simulink model "simulink_group17f"  (R2024a)
settings: Solver=FixedStepDiscrete  StartTime=0.0  StopTime=10.0  FixedStep=1e-3  RelTol=1e-3  EnableMultiTasking=on
undefined symbols (not defined in the file): A0, A1, D0, D1, D10, D11, D12, D13, D2, D3, D4, D5, D6, D7, D8, D9, PTA0, PTA1, PTA2, PTB2, PTB23, PTB3, PTB9, PTC16, PTC17, PTC2, PTC3, PTC4, PTD0, PTD1, PTD2, PTD3
libraries: frdmk64flib x20, dspstat3 x1, simulink x1
settings Model: ExtModeTrigDuration=5  Creator=ow  LastModifiedBy=furqa
settings SolverCC: AlgebraicLoopSolver=TrustRegion
settings OptimizationCC: EnhancedBackFolding=on  PassReuseOutputArgsAs=Individual arguments  ZeroExternalMemoryAtStartup=off  ZeroInternalMemoryAtStartup=off  MaxStackSize=64  OptimizeBlockOrder=speed  DifferentSizesBufferReuse=on  OptimizationCustomize=off  EfficientTunableParamExpr=on
settings DebuggingCC: ParameterTunabilityLossMsg=error  UnconnectedInputMsg=warning  UnconnectedOutputMsg=warning  UnconnectedLineMsg=warning
settings HardwareCC: ProdBitPerPointer=32  ProdBitPerSizeT=32  ProdBitPerPtrDiffT=32  ProdLargestAtomicInteger=Long  ProdLargestAtomicFloat=Double  ProdWordSize=32  ProdHWDeviceType=ARM Compatible->ARM Cortex
settings ModelReferenceCC: EnableRefExpFcnMdlSchedulingChecks=on
settings SFSimCC: MATLABDynamicMemAlloc=off
settings RTWCC: Description=Embedded Coder  SystemTargetFile=ert.tlc  HardwareBoard=NXP FRDM-K64F  TLCOptions="-aInlineSetEventsForThisBaseRateFcn=TLC_FALSE -aSuppressMultiTaskScheduler=TLC_FALSE  -aRateBasedStepFcn=0"  TemplateMakefile=ert_default_tmf  Toolchain=GNU Tools for ARM Embedded Processors  GPUComputeCapability=3.5
settings CodeAppCC: ForceParamTrailComments=on  IgnoreCustomStorageClasses=off  OperatorAnnotations=on  SimulinkDataObjDesc=on  SFDataObjDesc=on  InsertBlockDesc=on

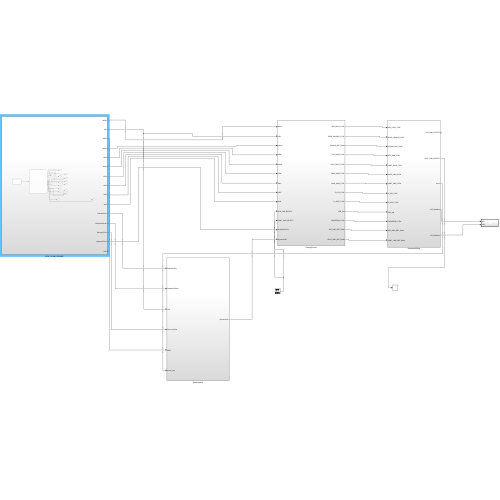
[thumbnail: Simulink's stored preview of the top-level diagram]
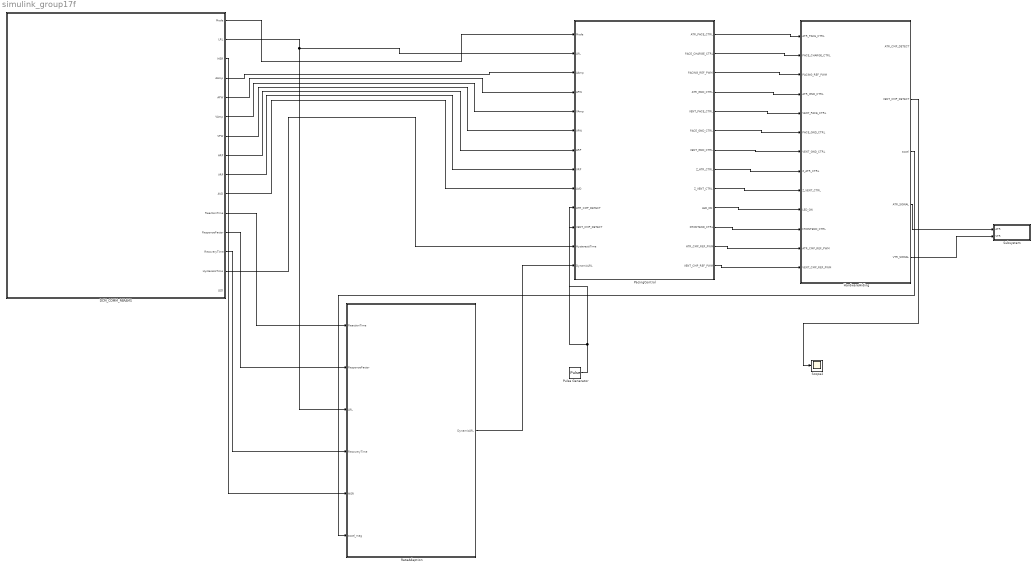
== system simulink_group17f ==
  DCM_COMM_PARAMS : Subsystem
  HardwareHiding : Subsystem
  PacingControl : Subsystem
  Pulse Generator : DiscretePulseGenerator  Period=600  PulseWidth=5  SampleTime=0.001
  RateAdaption : Subsystem
  Scope2 : Scope
  Subsystem : Subsystem  TreatAsAtomicUnit=on  SystemSampleTime=0.01
  wires:
  HardwareHiding/3(accel) -> RateAdaption/6(accel_mag)
  PacingControl/1(ATR_PACE_CTRL) -> HardwareHiding/1(ATR_PACE_CTRL)
  PacingControl/2(PACE_CHARGE_CTRL) -> HardwareHiding/2(PACE_CHARGE_CTRL)
  PacingControl/3(PACING_REF_PWM) -> HardwareHiding/3(PACING_REF_PWM)
  PacingControl/4(ATR_GND_CTRL) -> HardwareHiding/4(ATR_GND_CTRL)
  PacingControl/5(VENT_PACE_CTRL) -> HardwareHiding/5(VENT_PACE_CTRL)
  PacingControl/6(PACE_GND_CTRL) -> HardwareHiding/6(PACE_GND_CTRL)
  PacingControl/7(VENT_GND_CTRL) -> HardwareHiding/7(VENT_GND_CTRL)
  PacingControl/8(Z_ATR_CTRL) -> HardwareHiding/8(Z_ATR_CTRL)
  PacingControl/9(Z_VENT_CTRL) -> HardwareHiding/9(Z_VENT_CTRL)
  PacingControl/10(LED_ON) -> HardwareHiding/10(LED_ON)
  PacingControl/11(FRONTEND_CTRL) -> HardwareHiding/11(FRONTEND_CTRL)
  PacingControl/12(ATR_CMP_REF_PWM) -> HardwareHiding/12(ATR_CMP_REF_PWM)
  PacingControl/13(VENT_CMP_REF_PWM) -> HardwareHiding/13(VENT_CMP_REF_PWM)
  RateAdaption/1(DynamicLRL) -> PacingControl/13(DynamicLRL)
  HardwareHiding/2(VENT_CMP_DETECT) -> Scope2/1
  Pulse Generator/1 -> PacingControl/10(ATR_CMP_DETECT), PacingControl/11(VENT_CMP_DETECT)
  DCM_COMM_PARAMS/1(Mode) -> PacingControl/1(Mode)
  DCM_COMM_PARAMS/2(LRL) -> RateAdaption/3(LRL), PacingControl/2(LRL)
  DCM_COMM_PARAMS/3(MSR) -> RateAdaption/5(MSR)
  DCM_COMM_PARAMS/4(AAmp) -> PacingControl/3(AAmp)
  DCM_COMM_PARAMS/5(APW) -> PacingControl/4(APW)
  DCM_COMM_PARAMS/6(VAmp) -> PacingControl/5(VAmp)
  DCM_COMM_PARAMS/7(VPW) -> PacingControl/6(VPW)
  DCM_COMM_PARAMS/8(ARP) -> PacingControl/7(ARP)
  DCM_COMM_PARAMS/9(VRP) -> PacingControl/8(VRP)
  DCM_COMM_PARAMS/10(AVD) -> PacingControl/9(AVD)
  DCM_COMM_PARAMS/14(HysteresisTime) -> PacingControl/12(HysteresisTime)
  DCM_COMM_PARAMS/11(ReactionTime) -> RateAdaption/1(ReactionTime)
  DCM_COMM_PARAMS/12(ResponseFactor) -> RateAdaption/2(ResponseFactor)
  DCM_COMM_PARAMS/13(RecoveryTime) -> RateAdaption/4(RecoveryTime)
  HardwareHiding/4(ATR_SIGNAL) -> Subsystem/1(ATR)
  HardwareHiding/5(VTR_SIGNAL) -> Subsystem/2(VTR)

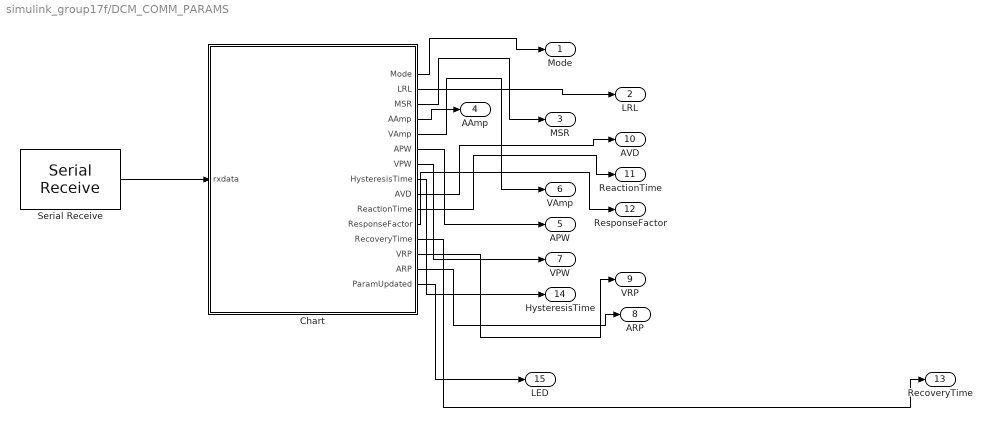
== system simulink_group17f/DCM_COMM_PARAMS ==
  Chart : Stateflow chart  TreatAsAtomicUnit=on
  Serial Receive : frdmk64flib/Serial Receive  SCIModule=0  Baudrate=uint32(9600)  Parity=None  StopBits=1  HardwareFlowControl=None  ByteOrder=LittleEndian  DataType=uint8  DataLength=31  BlockingMode=off  OutputStatus=off  SampleTime=0.001
  Mode : Outport
  LRL : Outport  Port=2
  MSR : Outport  Port=3
  AAmp : Outport  Port=4
  APW : Outport  Port=5
  VAmp : Outport  Port=6
  VPW : Outport  Port=7
  ARP : Outport  Port=8
  VRP : Outport  Port=9
  AVD : Outport  Port=10
  ReactionTime : Outport  Port=11
  ResponseFactor : Outport  Port=12
  RecoveryTime : Outport  Port=13
  HysteresisTime : Outport  Port=14
  LED : Outport  Port=15
  wires:
  Chart/1(Mode) -> Mode/1
  Chart/3(MSR) -> MSR/1
  Chart/4(AAmp) -> AAmp/1
  Chart/5(VAmp) -> VAmp/1
  Chart/6(APW) -> APW/1
  Chart/7(VPW) -> VPW/1
  Chart/8(HysteresisTime) -> HysteresisTime/1
  Chart/9(AVD) -> AVD/1
  Chart/10(ReactionTime) -> ReactionTime/1
  Chart/11(ResponseFactor) -> ResponseFactor/1
  Chart/13(VRP) -> VRP/1
  Chart/14(ARP) -> ARP/1
  Chart/2(LRL) -> LRL/1
  Chart/12(RecoveryTime) -> RecoveryTime/1
  Serial Receive/1 -> Chart/1(rxdata)
  Chart/15(ParamUpdated) -> LED/1

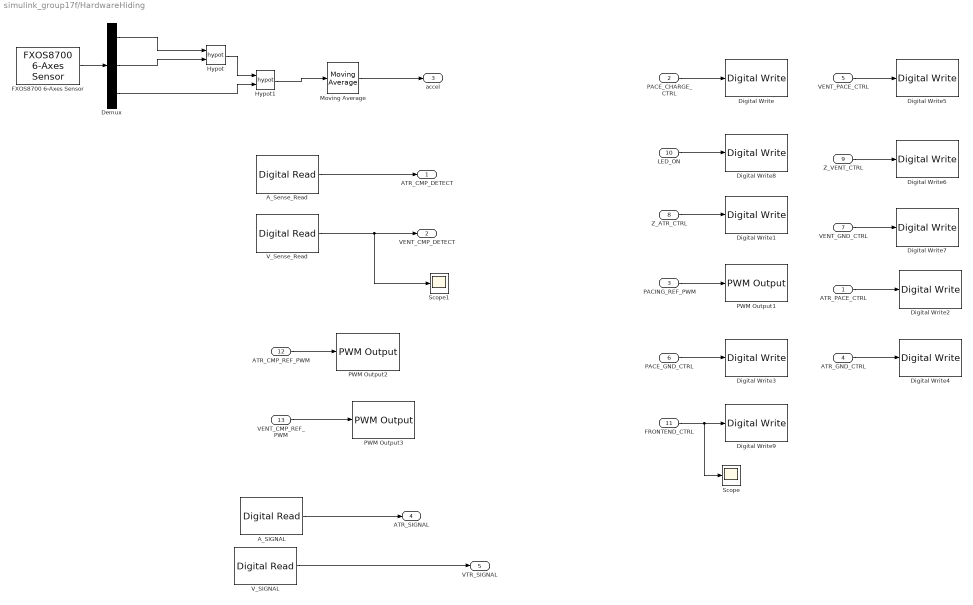
== system simulink_group17f/HardwareHiding ==
  ATR_PACE_CTRL : Inport
  PACE_CHARGE_CTRL : Inport  Port=2
  PACING_REF_PWM : Inport  Port=3
  ATR_GND_CTRL : Inport  Port=4
  VENT_PACE_CTRL : Inport  Port=5
  PACE_GND_CTRL : Inport  Port=6
  VENT_GND_CTRL : Inport  Port=7
  Z_ATR_CTRL : Inport  Port=8
  Z_VENT_CTRL : Inport  Port=9
  LED_ON : Inport  Port=10
  FRONTEND_CTRL : Inport  Port=11
  ATR_CMP_REF_PWM : Inport  Port=12
  VENT_CMP_REF_PWM : Inport  Port=13
  A_SIGNAL : frdmk64flib/Digital Read  Whichpin=PTB2 (A0)  SampleTime=0.01
  A_Sense_Read : frdmk64flib/Digital Read  Whichpin=PTC16 (D0)  SampleTime=-1
  Demux : Demux  Outputs=3
  Digital Write : frdmk64flib/Digital Write  Whichpin=PTB9 (D2)
  Digital Write1 : frdmk64flib/Digital Write  Whichpin=PTB23 (D4)
  Digital Write2 : frdmk64flib/Digital Write  Whichpin=PTA0 (D8)
  Digital Write3 : frdmk64flib/Digital Write  Whichpin=PTD0 (D10)
  Digital Write4 : frdmk64flib/Digital Write  Whichpin=PTD2 (D11)
  Digital Write5 : frdmk64flib/Digital Write  Whichpin=PTC4 (D9)
  Digital Write6 : frdmk64flib/Digital Write  Whichpin=PTC3 (D7)
  Digital Write7 : frdmk64flib/Digital Write  Whichpin=PTD3 (D12)
  Digital Write8 : frdmk64flib/Digital Write  Whichpin=RED_LED
  Digital Write9 : frdmk64flib/Digital Write  Whichpin=PTD1 (D13)
  FXOS8700 6-Axes Sensor : frdmk64flib/FXOS8700 6-Axes Sensor  Activesensor=Accelerometer only  ODR=800Hz  HybridODR=400Hz  Accelfullrange=-4g to +4g  SampleTime=-1
  Hypot : Math  Operator=hypot
  Hypot1 : Math  Operator=hypot
  Moving Average : dspstat3/Moving Average  Method=Sliding window  ForgettingFactorPort=off  SpecifyWindowLength=on  WindowLength=4  OverlapLength=3  AllowArbitraryInputLength=off  ForgettingFactor=0.9  SimulateUsing=Interpreted execution
  PWM Output1 : frdmk64flib/PWM Output  Whichpin=PTA2 (D5)  InitialFrequency=2000  InitialDutyCycle=50
  PWM Output2 : frdmk64flib/PWM Output  Whichpin=PTC2 (D6)  InitialFrequency=2000  InitialDutyCycle=100
  PWM Output3 : frdmk64flib/PWM Output  Whichpin=PTA1 (D3)  InitialFrequency=2000  InitialDutyCycle=100
  Scope : Scope
  Scope1 : Scope
  V_SIGNAL : frdmk64flib/Digital Read  Whichpin=PTB3 (A1)  SampleTime=0.01
  V_Sense_Read : frdmk64flib/Digital Read  Whichpin=PTC17 (D1)  SampleTime=-1
  ATR_CMP_DETECT : Outport
  VENT_CMP_DETECT : Outport  Port=2
  accel : Outport  Port=3
  ATR_SIGNAL : Outport  Port=4
  VTR_SIGNAL : Outport  Port=5
  wires:
  V_Sense_Read/1 -> Scope1/1, VENT_CMP_DETECT/1
  Z_VENT_CTRL/1 -> Digital Write6/1
  LED_ON/1 -> Digital Write8/1
  ATR_PACE_CTRL/1 -> Digital Write2/1
  Z_ATR_CTRL/1 -> Digital Write1/1
  VENT_GND_CTRL/1 -> Digital Write7/1
  PACE_CHARGE_CTRL/1 -> Digital Write/1
  PACE_GND_CTRL/1 -> Digital Write3/1
  PACING_REF_PWM/1 -> PWM Output1/1
  VENT_PACE_CTRL/1 -> Digital Write5/1
  ATR_GND_CTRL/1 -> Digital Write4/1
  FRONTEND_CTRL/1 -> Scope/1, Digital Write9/1
  ATR_CMP_REF_PWM/1 -> PWM Output2/1
  VENT_CMP_REF_PWM/1 -> PWM Output3/1
  Demux/1 -> Hypot/1
  Demux/2 -> Hypot/2
  Hypot/1 -> Hypot1/1
  Demux/3 -> Hypot1/2
  Hypot1/1 -> Moving Average/1
  Moving Average/1 -> accel/1
  A_Sense_Read/1 -> ATR_CMP_DETECT/1
  FXOS8700 6-Axes Sensor/1 -> Demux/1
  A_SIGNAL/1 -> ATR_SIGNAL/1
  V_SIGNAL/1 -> VTR_SIGNAL/1

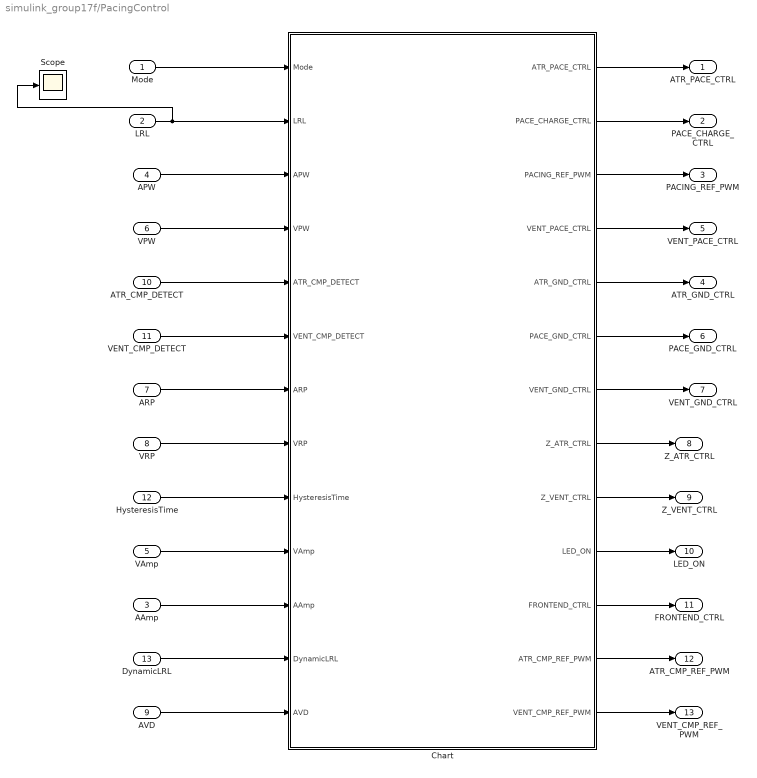
== system simulink_group17f/PacingControl ==
  Mode : Inport
  LRL : Inport  Port=2
  AAmp : Inport  Port=3
  APW : Inport  Port=4
  VAmp : Inport  Port=5
  VPW : Inport  Port=6
  ARP : Inport  Port=7
  VRP : Inport  Port=8
  AVD : Inport  Port=9
  ATR_CMP_DETECT : Inport  Port=10
  VENT_CMP_DETECT : Inport  Port=11
  HysteresisTime : Inport  Port=12
  DynamicLRL : Inport  Port=13
  Chart : Stateflow chart  TreatAsAtomicUnit=on
      settings: PortSchema="{\"entries\":[{\"content\":{\"sides\":[{\"content\":{\"connectorIds\":[\"In1\",\"In2\",\"In5\",\"In3\",\"In4\",\"In6\",\"In7\",\"In10\",\"In11\",\"In8\",\"In9\",\"In12\",\"In13\"]},\"type\":\"ConnectorPlacement.EquallySpacedRectSide\",\"uuid\":\"2cabd690-10ca-439e-b217-62815d125176\"},{\"content\":{\"connectorIds\":[\"Out1\",\"Out2\",\"Out3\",\"Out4\",\"Out5\",\"Out6\",\"Out7\",\"Out8\",\"Out9\",\"Out10\",\"Out11\",\"Out12\",\"Out13\"],\"side\":\"RIGHT\"},\"type\":\"ConnectorPlacement.EquallySpacedRectSide\",\"uuid\":\"e8964e9d-7b02-47f5-a48a-30c87640778e\"},{\"content\":{\"side\":\"TOP\"},\"type\":\"ConnectorPlacement.EquallySpacedRectSide\",\"uuid\":\"37da63f5-52a1-4b9c-b728-2e179414b5fa\"}]},\"type\":\"ConnectorPlacement.EquallySpacedConnector\",\"uuid\":\"fe4480b5-e88f-4b9f-8d05-cd2d47a8a31d\"}],\"packageUris\":[\"http://schema.mathworks.com/mf0/Connector/R2020b\"],\"version\":\"1.0\"}"
  Scope : Scope
  ATR_PACE_CTRL : Outport
  PACE_CHARGE_CTRL : Outport  Port=2
  PACING_REF_PWM : Outport  Port=3
  ATR_GND_CTRL : Outport  Port=4
  VENT_PACE_CTRL : Outport  Port=5
  PACE_GND_CTRL : Outport  Port=6
  VENT_GND_CTRL : Outport  Port=7
  Z_ATR_CTRL : Outport  Port=8
  Z_VENT_CTRL : Outport  Port=9
  LED_ON : Outport  Port=10
  FRONTEND_CTRL : Outport  Port=11
  ATR_CMP_REF_PWM : Outport  Port=12
  VENT_CMP_REF_PWM : Outport  Port=13
  wires:
  Mode/1 -> Chart/1(Mode)
  VPW/1 -> Chart/3(VPW)
  ATR_CMP_DETECT/1 -> Chart/4(ATR_CMP_DETECT)
  APW/1 -> Chart/5(APW)
  ARP/1 -> Chart/7(ARP)
  VRP/1 -> Chart/10(VRP)
  AAmp/1 -> Chart/9(AAmp)
  VAmp/1 -> Chart/8(VAmp)
  Chart/1(ATR_PACE_CTRL) -> ATR_PACE_CTRL/1
  Chart/2(PACE_CHARGE_CTRL) -> PACE_CHARGE_CTRL/1
  Chart/3(PACING_REF_PWM) -> PACING_REF_PWM/1
  Chart/5(ATR_GND_CTRL) -> ATR_GND_CTRL/1
  Chart/6(PACE_GND_CTRL) -> PACE_GND_CTRL/1
  Chart/7(VENT_GND_CTRL) -> VENT_GND_CTRL/1
  Chart/8(Z_ATR_CTRL) -> Z_ATR_CTRL/1
  Chart/9(Z_VENT_CTRL) -> Z_VENT_CTRL/1
  Chart/11(FRONTEND_CTRL) -> FRONTEND_CTRL/1
  HysteresisTime/1 -> Chart/11(HysteresisTime)
  Chart/4(VENT_PACE_CTRL) -> VENT_PACE_CTRL/1
  Chart/10(LED_ON) -> LED_ON/1
  VENT_CMP_DETECT/1 -> Chart/6(VENT_CMP_DETECT)
  Chart/12(ATR_CMP_REF_PWM) -> ATR_CMP_REF_PWM/1
  Chart/13(VENT_CMP_REF_PWM) -> VENT_CMP_REF_PWM/1
  AVD/1 -> Chart/13(AVD)
  LRL/1 -> Scope/1, Chart/2(LRL)
  DynamicLRL/1 -> Chart/12(DynamicLRL)

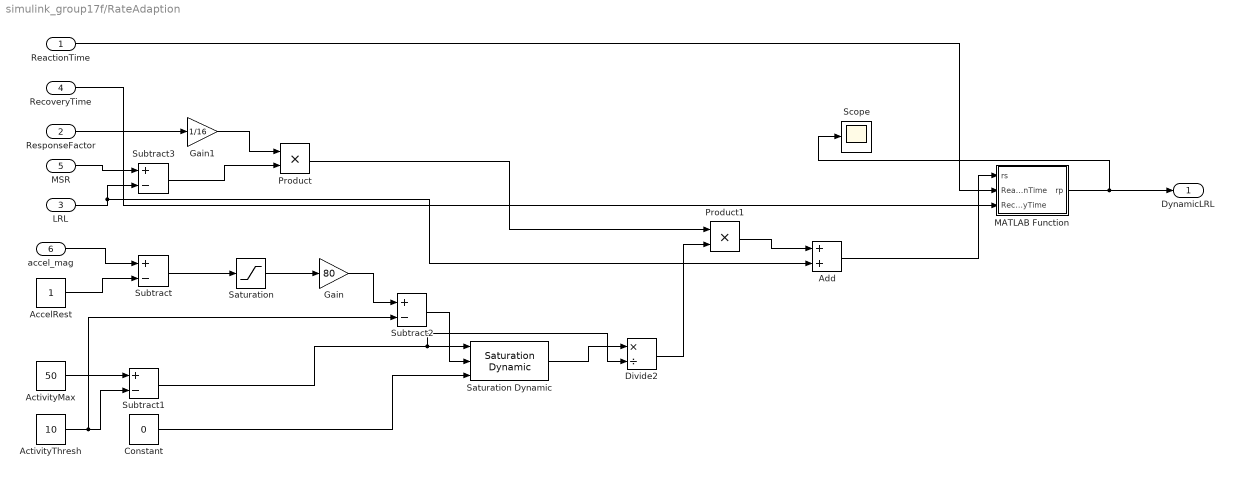
== system simulink_group17f/RateAdaption ==
  ReactionTime : Inport
  ResponseFactor : Inport  Port=2
  LRL : Inport  Port=3
  RecoveryTime : Inport  Port=4
  MSR : Inport  Port=5
  accel_mag : Inport  Port=6
  AccelRest : Constant
  ActivityMax : Constant  Value=50
  ActivityThresh : Constant  Value=10
  Add : Sum
  Constant : Constant  Value=0
  Divide2 : Product  Inputs=*/
  Gain : Gain  Gain=80
  Gain1 : Gain  Gain=1/16
  MATLAB Function : MATLAB Function  TreatAsAtomicUnit=on
  Product : Product
  Product1 : Product
  Saturation : Saturate  UpperLimit=1  LowerLimit=0
  Saturation Dynamic : simulink/Discontinuities/Saturation Dynamic  OutMin=[]  OutMax=[]  OutDataTypeStr=Inherit: Same as second input  OutDataType=fixdt(1, 16)  OutScaling=2^-10  DoSatur=off
  Scope : Scope
  Subtract{,1..3} (4 alike) : Sum  Inputs=+-
  DynamicLRL : Outport
  wires:
  accel_mag/1 -> Subtract/1
  AccelRest/1 -> Subtract/2
  Subtract/1 -> Saturation/1
  Saturation/1 -> Gain/1
  ActivityMax/1 -> Subtract1/1
  Subtract1/1 -> Divide2/2, Saturation Dynamic/1
  Gain/1 -> Subtract2/1
  Subtract2/1 -> Saturation Dynamic/2
  Constant/1 -> Saturation Dynamic/3
  ActivityThresh/1 -> Subtract2/2, Subtract1/2
  ResponseFactor/1 -> Gain1/1
  MSR/1 -> Subtract3/1
  LRL/1 -> Add/2, Subtract3/2
  Saturation Dynamic/1 -> Divide2/1
  Gain1/1 -> Product/1
  Subtract3/1 -> Product/2
  Divide2/1 -> Product1/2
  Product/1 -> Product1/1
  Product1/1 -> Add/1
  ReactionTime/1 -> MATLAB Function/2(ReactionTime)
  RecoveryTime/1 -> MATLAB Function/3(RecoveryTime)
  MATLAB Function/1(rp) -> Scope/1, DynamicLRL/1
  Add/1 -> MATLAB Function/1(rs)

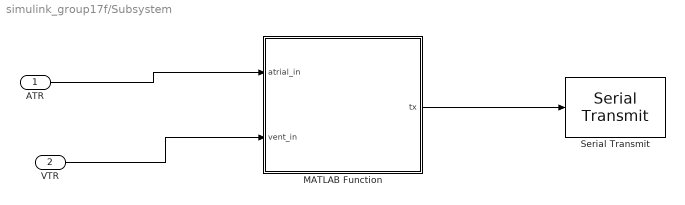
== system simulink_group17f/Subsystem ==
  ATR : Inport
  VTR : Inport  Port=2
  MATLAB Function : MATLAB Function  TreatAsAtomicUnit=on
  Serial Transmit : frdmk64flib/Serial Transmit  SCIModule=0  Baudrate=uint32(9600)  Parity=None  StopBits=1  HardwareFlowControl=None  ByteOrder=LittleEndian  BlockingMode=off  OutputStatus=off
  wires:
  ATR/1 -> MATLAB Function/1(atrial_in)
  VTR/1 -> MATLAB Function/2(vent_in)
  MATLAB Function/1(tx) -> Serial Transmit/1

== stateflow chart simulink_group17f/DCM_COMM_PARAMS/Chart ==
  state INITIAL_
    % Set initial values of parameters
    Mode = 1;
    LRL = 60;
    MSR = 120;
    AAmp = 3.5;
    VAmp = 3.5;
    APW = 0.4;
    VPW = 0.4;
    VRP = 320;
    ARP = 250;
    HysteresisTime = 1;
    AVD = 150;
    ReactionTime = 3;   % Seconds
    ResponseFactor = 8;  % factor 1-16
    RecoveryTime = 5;    % seconds
  state SET_PARAM_
    % 1-byte fields → just cast to double
    % Basic structural checks
    ParamUpdated = false;
    if length(rxdata) < 31
    % Not enough bytes – ignore
    return;
    end
    % Optional: header + length check
    if rxdata(2) ~= 0
    % Wrong header or length – ignore
    return;
    end
    Mode = double(rxdata(3));
    LRL  = double(rxdata(4));
    MSR  = double(rxdata(5));   % if you actually need MSR
    % 4-byte floats → typecast then convert to double
    tmpAAmp = zeros(1,4);
    tmpAAmp(1) = typecast(uint8(rxdata(6:9)), 'single');
    AAmp = double(tmpAAmp(1));
    tmpVAmp = zeros(1,4);
    tmpVAmp(1) = typecast(uint8(rxdata(10:13)), 'single');
    VAmp = double(tmpVAmp(1));
    tmpAPW = zeros(1,4);
    tmpAPW(1) = typecast(uint8(rxdata(14:17)), 'single');
    APW = double(tmpAPW(1));
    tmpVPW = zeros(1,4);
    tmpVPW(1) = typecast(uint8(rxdata(18:21)), 'single');
    VPW = double(tmpVPW(1));
    % 2-byte ints → typecast then convert to double
    tmpVRP = zeros(1,2);
    tmpVRP(1) = typecast(uint8(rxdata(22:23)), 'uint16');
    VRP = double(tmpVRP(1));
    tmpARP = zeros(1,2);
    tmpARP(1) = typecast(uint8(rxdata(24:25)), 'uint16');
    ARP = double(tmpARP(1));
    % Remaining 1-byte fields → cast to double
    HysteresisTime   = double(rxdata(26));
    % 2-byte ints → typecast then convert to double
    tmpAVD = zeros(1,2);
    tmpAVD(1) = typecast(uint8(rxdata(27:28)), 'uint16');
    AVD = double(tmpAVD(1));
    % Remaining 1-byte fields → cast to double
    ReactionTime     = double(rxdata(29));   % seconds/minutes
    ResponseFactor   = double(rxdata(30));
    RecoveryTime    = double(rxdata(31));
    % initialize to zero (required by Stateflow)
    %echoBuffer = uint8(zeros(1,31));
    %for i = 1:31
    % echoBuffer(i) = rxdata(i);
    %end
    send_params();
    ParamUpdated = true;
  state WAIT_FRAME
  state ECHO_PARAM
    entry:
    send_params();
  (default) -> INITIAL_
  INITIAL_ -> WAIT_FRAME : after(0.1,sec)
  WAIT_FRAME -> SET_PARAM_ : [[rxdata(1) == 1]]
  SET_PARAM_ -> ECHO_PARAM
  data: rxdata input uint8 size=31; Mode output double size=1; LRL output double size=1; MSR output double size=1; AAmp output double size=1; VAmp output double size=1; APW output double size=1; VPW output double size=1; HysteresisTime output double size=1; AVD output double size=1; ReactionTime output double size=1; ResponseFactor output double size=1; RecoveryTime output double size=1; VRP output double size=1; ARP output double size=1; tmpAAmp local; tmpAPW local; tmpVAmp local; tmpARP local; tmpVRP local; tmpVPW local; tmpAVD local; dummy local; i local; ParamUpdated output
  function send_params:
    | function send_params()
    | % TODO: implement UART / serial TX using Simulink interfaces
    | end

== matlab function simulink_group17f/RateAdaption/MATLAB Function ==
  data: rs input; ReactionTime input; RecoveryTime input; rp output
function rp = timeResponse(rs, ReactionTime, RecoveryTime)
persistent currentRate
if isempty(currentRate)
    currentRate = rs; 
end

dt = 0.01;

if rs > currentRate
   
    if ReactionTime <= 0
        alpha = 1;
    else
        alpha = dt / ReactionTime;
    end
elseif rs < currentRate
   
    if RecoveryTime <= 0
        alpha = 1;
    else
        alpha = dt / RecoveryTime;
    end
else
    alpha = 0;
end


if alpha > 1
    alpha = 1;
elseif alpha < 0
    alpha = 0;
end

currentRate = currentRate + alpha * (rs - currentRate);
rp = currentRate;

== stateflow chart simulink_group17f/PacingControl/Chart ==
  state AOO
    state APacing
      entry:
      %Pace Atrial
      PACE_CHARGE_CTRL = 0;
      PACE_GND_CTRL = 1;
      ATR_PACE_CTRL = 1;
      ATR_GND_CTRL = 0;
      VENT_PACE_CTRL = 0;
      VENT_GND_CTRL = 0;
      Z_ATR_CTRL = 0;
      Z_VENT_CTRL = 0;
      LED_ON = 1;
    state ChargingDischarging
      entry:
      %No Sensing
      FRONTEND_CTRL = 0;
      %Charging
      PACE_CHARGE_CTRL = 1;
      ATR_PACE_CTRL = 0;
      VENT_PACE_CTRL = 0;
      PACING_REF_PWM = (AAmp/5) * 100;
      %Discharging
      PACE_GND_CTRL = 1;
      ATR_PACE_CTRL = 0;
      ATR_GND_CTRL = 1;
      VENT_PACE_CTRL = 0;
      VENT_GND_CTRL = 0;
      Z_ATR_CTRL = 0;
      Z_VENT_CTRL = 0;
      LED_ON = 0;
    (default) -> state26
    AOO.APacing -> state26 : [after(APW,msec)]
    state26 -> AOO.APacing : [after((60000/double(LRL))-APW,msec)]
  state VOO
    state Chargin_Discharging
      entry:
      %No Sensing
      FRONTEND_CTRL = 0;
      %Charging
      PACE_CHARGE_CTRL = 1;
      ATR_PACE_CTRL = 0;
      VENT_PACE_CTRL = 0;
      PACING_REF_PWM = (VAmp/5) * 100;
      %Discharging
      PACE_GND_CTRL = 1;
      ATR_PACE_CTRL = 0;
      ATR_GND_CTRL = 0;
      VENT_PACE_CTRL = 0;
      VENT_GND_CTRL = 1;
      Z_ATR_CTRL = 0;
      Z_VENT_CTRL = 0;
      LED_ON = 0;
    state Pacing
      entry:
      %Pace Ventricle
      PACE_CHARGE_CTRL = 0;
      PACE_GND_CTRL = 1;
      ATR_PACE_CTRL = 0;
      ATR_GND_CTRL = 0;
      VENT_PACE_CTRL = 1;
      VENT_GND_CTRL = 0;
      Z_ATR_CTRL = 0;
      Z_VENT_CTRL = 0;
      LED_ON = 1;
    (default) -> VOO.Chargin_Discharging
    VOO.Chargin_Discharging -> VOO.Pacing : [after((60000/double(LRL))-VPW,msec)]
    VOO.Pacing -> VOO.Chargin_Discharging : [after(VPW,msec)]
  state AAI
    state ChargingDischarging
      entry:
      %Enable Sensing
      FRONTEND_CTRL = 1;
      ATR_CMP_REF_PWM = 90;
      %Charging
      PACE_CHARGE_CTRL = 1;
      ATR_PACE_CTRL = 0;
      VENT_PACE_CTRL = 0;
      PACING_REF_PWM = (AAmp/5) * 100;
      %Discharging
      PACE_GND_CTRL = 1;
      ATR_PACE_CTRL = 0;
      ATR_GND_CTRL = 1;
      VENT_PACE_CTRL = 0;
      VENT_GND_CTRL = 0;
      Z_ATR_CTRL = 0;
      Z_VENT_CTRL = 0;
      LED_ON = 0;
    state Pacing
      entry:
      %Disable Sensing
      FRONTEND_CTRL = 0;
      %Pace Ventricle
      PACE_CHARGE_CTRL = 0;
      PACE_GND_CTRL = 1;
      ATR_PACE_CTRL = 1;
      ATR_GND_CTRL = 0;
      VENT_PACE_CTRL = 0;
      VENT_GND_CTRL = 0;
      Z_ATR_CTRL = 0;
      Z_VENT_CTRL = 0;
      LED_ON = 1;
    state Hysteresis
      entry:
      %Enable Sensing
      FRONTEND_CTRL = 1;
      %Charging
      PACE_CHARGE_CTRL = 1;
      ATR_PACE_CTRL = 0;
      VENT_PACE_CTRL = 0;
      %Discharging
      PACE_GND_CTRL = 1;
      ATR_PACE_CTRL = 0;
      ATR_GND_CTRL = 1;
      VENT_PACE_CTRL = 0;
      VENT_GND_CTRL = 0;
      Z_ATR_CTRL = 0;
      Z_VENT_CTRL = 0;
      LED_ON = 0;
    (default) -> AAI.ChargingDischarging
    AAI.ChargingDischarging -> AAI.Pacing [order 1] : [after(double(60000/LRL)- ARP, msec) ]
    AAI.Pacing -> AAI.ChargingDischarging : [after(APW,msec)]
    AAI.Hysteresis -> AAI.Pacing [order 2] : [after(double(60000/LRL) + HysteresisTime, msec)]
    AAI.Hysteresis -> AAI.ChargingDischarging [order 3] : [after(ARP, msec)]
    AAI.ChargingDischarging -> AAI.Hysteresis [order 2] : [ ATR_CMP_DETECT==1]
    AAI.Hysteresis -> AAI.Hysteresis [order 1] : [after(ARP, msec) && ATR_CMP_DETECT==1]
  state VVI
    state ChargingDischarging
      entry:
      %Enable Sensing
      FRONTEND_CTRL = 1;
      VENT_CMP_REF_PWM = 90;
      %Charging
      PACE_CHARGE_CTRL = 1;
      ATR_PACE_CTRL = 0;
      VENT_PACE_CTRL = 0;
      PACING_REF_PWM = (VAmp/5) * 100;
      %Discharging
      PACE_GND_CTRL = 1;
      ATR_PACE_CTRL = 0;
      ATR_GND_CTRL = 0;
      VENT_PACE_CTRL = 0;
      VENT_GND_CTRL = 1;
      Z_ATR_CTRL = 0;
      Z_VENT_CTRL = 0;
      LED_ON = 0;
    state VPacing
      entry:
      %Disable Sensing
      FRONTEND_CTRL = 0;
      %Pace Ventricle
      PACE_CHARGE_CTRL = 0;
      PACE_GND_CTRL = 1;
      ATR_PACE_CTRL = 0;
      ATR_GND_CTRL = 0;
      VENT_PACE_CTRL = 1;
      VENT_GND_CTRL = 0;
      Z_ATR_CTRL = 0;
      Z_VENT_CTRL = 0;
      LED_ON = 1;
    state Hysteresis
      entry:
      %Enable Sensing
      FRONTEND_CTRL = 1;
      %Charging
      PACE_CHARGE_CTRL = 1;
      ATR_PACE_CTRL = 0;
      VENT_PACE_CTRL = 0;
      %Discharging
      PACE_GND_CTRL = 1;
      ATR_PACE_CTRL = 0;
      ATR_GND_CTRL = 0;
      VENT_PACE_CTRL = 0;
      VENT_GND_CTRL = 1;
      Z_ATR_CTRL = 0;
      Z_VENT_CTRL = 0;
      LED_ON = 0;
    (default) -> VVI.ChargingDischarging
    VVI.ChargingDischarging -> VVI.VPacing [order 1] : [after(double(60000/LRL)-VRP, msec) ]
    VVI.VPacing -> VVI.ChargingDischarging : [after(VPW,msec)]
    VVI.Hysteresis -> VVI.VPacing [order 2] : [after(double(60000/LRL) + HysteresisTime, msec)]
    VVI.Hysteresis -> VVI.ChargingDischarging [order 3] : [after(VRP, msec)]
    VVI.ChargingDischarging -> VVI.Hysteresis [order 2] : [ VENT_CMP_DETECT==1]
    VVI.Hysteresis -> VVI.Hysteresis [order 1] : [after(VRP, msec) && VENT_CMP_DETECT==1]
  state DDDR
    state Apace
      entry:
      %Disable Sensing
      FRONTEND_CTRL = 0;
      %Pace Ventricle
      PACE_CHARGE_CTRL = 0;
      PACE_GND_CTRL = 1;
      ATR_PACE_CTRL = 1;
      ATR_GND_CTRL = 0;
      VENT_PACE_CTRL = 0;
      VENT_GND_CTRL = 0;
      Z_ATR_CTRL = 0;
      Z_VENT_CTRL = 0;
      LED_ON = 1;
    state Await
      entry:
      %Enable Sensing
      FRONTEND_CTRL = 1;
      ATR_CMP_REF_PWM = 90;
      %Charging
      PACE_CHARGE_CTRL = 1;
      ATR_PACE_CTRL = 0;
      VENT_PACE_CTRL = 0;
      PACING_REF_PWM = (AAmp/5) * 100;
      %Discharging
      PACE_GND_CTRL = 1;
      ATR_PACE_CTRL = 0;
      ATR_GND_CTRL = 1;
      VENT_PACE_CTRL = 0;
      VENT_GND_CTRL = 0;
      Z_ATR_CTRL = 0;
      Z_VENT_CTRL = 0;
      LED_ON = 0;
    state AV_Wait
      entry:
      %Enable Sensing
      FRONTEND_CTRL = 1;
      VENT_CMP_REF_PWM = 90;
      %Charging
      PACE_CHARGE_CTRL = 1;
      ATR_PACE_CTRL = 0;
      VENT_PACE_CTRL = 0;
      PACING_REF_PWM = (VAmp/5) * 100;
      %Discharging
      PACE_GND_CTRL = 1;
      ATR_PACE_CTRL = 0;
      ATR_GND_CTRL = 0;
      VENT_PACE_CTRL = 0;
      VENT_GND_CTRL = 1;
      Z_ATR_CTRL = 0;
      Z_VENT_CTRL = 0;
      LED_ON = 0;
    state VPacing
      entry:
      %Disable Sensing
      FRONTEND_CTRL = 0;
      %Pace Ventricle
      PACE_CHARGE_CTRL = 0;
      PACE_GND_CTRL = 1;
      ATR_PACE_CTRL = 0;
      ATR_GND_CTRL = 0;
      VENT_PACE_CTRL = 1;
      VENT_GND_CTRL = 0;
      Z_ATR_CTRL = 0;
      Z_VENT_CTRL = 0;
      LED_ON = 1;
    (default) -> Await
    Await -> Apace [order 2] : [after(double(60000/DynamicLRL), msec)]
    Apace -> AV_Wait : [after(APW, msec)]
    Await -> AV_Wait [order 1] : [ATR_CMP_DETECT == 1]
    DDDR.VPacing -> Await : [after(VPW, msec)]
    AV_Wait -> Await [order 1] : [VENT_CMP_DETECT == 1]
    AV_Wait -> DDDR.VPacing [order 2] : [after(AVD, msec)]
  state InitialState
  state VVIR
    state ChargingDischarging
      entry:
      %Enable Sensing
      FRONTEND_CTRL = 1;
      VENT_CMP_REF_PWM = 90;
      %Charging
      PACE_CHARGE_CTRL = 1;
      ATR_PACE_CTRL = 0;
      VENT_PACE_CTRL = 0;
      PACING_REF_PWM = (VAmp/5) * 100;
      %Discharging
      PACE_GND_CTRL = 1;
      ATR_PACE_CTRL = 0;
      ATR_GND_CTRL = 0;
      VENT_PACE_CTRL = 0;
      VENT_GND_CTRL = 1;
      Z_ATR_CTRL = 0;
      Z_VENT_CTRL = 0;
      LED_ON = 0;
    state VPacing
      entry:
      %Disable Sensing
      FRONTEND_CTRL = 0;
      %Pace Ventricle
      PACE_CHARGE_CTRL = 0;
      PACE_GND_CTRL = 1;
      ATR_PACE_CTRL = 0;
      ATR_GND_CTRL = 0;
      VENT_PACE_CTRL = 1;
      VENT_GND_CTRL = 0;
      Z_ATR_CTRL = 0;
      Z_VENT_CTRL = 0;
      LED_ON = 1;
    state Hysteresis
      entry:
      %Enable Sensing
      FRONTEND_CTRL = 1;
      %Charging
      PACE_CHARGE_CTRL = 1;
      ATR_PACE_CTRL = 0;
      VENT_PACE_CTRL = 0;
      %Discharging
      PACE_GND_CTRL = 1;
      ATR_PACE_CTRL = 0;
      ATR_GND_CTRL = 0;
      VENT_PACE_CTRL = 0;
      VENT_GND_CTRL = 1;
      Z_ATR_CTRL = 0;
      Z_VENT_CTRL = 0;
      LED_ON = 0;
    (default) -> VVIR.ChargingDischarging
    VVIR.ChargingDischarging -> VVIR.VPacing [order 1] : [after(double(60000/DynamicLRL)-VRP, msec)]
    VVIR.VPacing -> VVIR.ChargingDischarging : [after(VPW,msec)]
    VVIR.Hysteresis -> VVIR.VPacing [order 2] : [after(double(60000/DynamicLRL)+ HysteresisTime, msec)]
    VVIR.Hysteresis -> VVIR.ChargingDischarging [order 3] : [after(VRP, msec)]
    VVIR.ChargingDischarging -> VVIR.Hysteresis [order 2] : [ VENT_CMP_DETECT==1]
    VVIR.Hysteresis -> VVIR.Hysteresis [order 1] : [after(VRP, msec) && VENT_CMP_DETECT==1]
  state AOOR
    state ChargingDischarging
      entry:
      %No Sensing
      FRONTEND_CTRL = 0;
      %Charging
      PACE_CHARGE_CTRL = 1;
      ATR_PACE_CTRL = 0;
      VENT_PACE_CTRL = 0;
      PACING_REF_PWM = (AAmp/5) * 100;
      %Discharging
      PACE_GND_CTRL = 1;
      ATR_PACE_CTRL = 0;
      ATR_GND_CTRL = 1;
      VENT_PACE_CTRL = 0;
      VENT_GND_CTRL = 0;
      Z_ATR_CTRL = 0;
      Z_VENT_CTRL = 0;
      LED_ON = 0;
    state APacing
      entry:
      %Pace Atrial
      PACE_CHARGE_CTRL = 0;
      PACE_GND_CTRL = 1;
      ATR_PACE_CTRL = 1;
      ATR_GND_CTRL = 0;
      VENT_PACE_CTRL = 0;
      VENT_GND_CTRL = 0;
      Z_ATR_CTRL = 0;
      Z_VENT_CTRL = 0;
      LED_ON = 1;
    (default) -> AOOR.ChargingDischarging
    AOOR.APacing -> AOOR.ChargingDischarging : [after(APW,msec)]
    AOOR.ChargingDischarging -> AOOR.APacing : [after(double(60000/DynamicLRL)-APW,msec)]
  state AAIR
    state ChargingDischarging
      entry:
      %Enable Sensing
      FRONTEND_CTRL = 1;
      ATR_CMP_REF_PWM = 90;
      %Charging
      PACE_CHARGE_CTRL = 1;
      ATR_PACE_CTRL = 0;
      VENT_PACE_CTRL = 0;
      PACING_REF_PWM = (AAmp/5) * 100;
      %Discharging
      PACE_GND_CTRL = 1;
      ATR_PACE_CTRL = 0;
      ATR_GND_CTRL = 1;
      VENT_PACE_CTRL = 0;
      VENT_GND_CTRL = 0;
      Z_ATR_CTRL = 0;
      Z_VENT_CTRL = 0;
      LED_ON = 0;
    state Pacing
      entry:
      %Disable Sensing
      FRONTEND_CTRL = 0;
      %Pace Ventricle
      PACE_CHARGE_CTRL = 0;
      PACE_GND_CTRL = 1;
      ATR_PACE_CTRL = 1;
      ATR_GND_CTRL = 0;
      VENT_PACE_CTRL = 0;
      VENT_GND_CTRL = 0;
      Z_ATR_CTRL = 0;
      Z_VENT_CTRL = 0;
      LED_ON = 1;
    state Hysteresis
      entry:
      %Enable Sensing
      FRONTEND_CTRL = 1;
      %Charging
      PACE_CHARGE_CTRL = 1;
      ATR_PACE_CTRL = 0;
      VENT_PACE_CTRL = 0;
      %Discharging
      PACE_GND_CTRL = 1;
      ATR_PACE_CTRL = 0;
      ATR_GND_CTRL = 1;
      VENT_PACE_CTRL = 0;
      VENT_GND_CTRL = 0;
      Z_ATR_CTRL = 0;
      Z_VENT_CTRL = 0;
      LED_ON = 0;
    (default) -> AAIR.ChargingDischarging
    AAIR.ChargingDischarging -> AAIR.Pacing [order 1] : [after(double(60000/DynamicLRL)- ARP, msec) ]
    AAIR.Pacing -> AAIR.ChargingDischarging : [after(APW,msec)]
    AAIR.Hysteresis -> AAIR.Pacing [order 2] : [after(double(60000/DynamicLRL)+ HysteresisTime, msec)]
    AAIR.Hysteresis -> AAIR.ChargingDischarging [order 3] : [after(ARP, msec)]
    AAIR.ChargingDischarging -> AAIR.Hysteresis [order 2] : [ ATR_CMP_DETECT==1]
    AAIR.Hysteresis -> AAIR.Hysteresis [order 1] : [after(ARP, msec) && ATR_CMP_DETECT==1]
  state VOOR
    state Chargin_Discharging
      entry:
      %No Sensing
      FRONTEND_CTRL = 0;
      %Charging
      PACE_CHARGE_CTRL = 1;
      ATR_PACE_CTRL = 0;
      VENT_PACE_CTRL = 0;
      PACING_REF_PWM = (VAmp/5) * 100;
      %Discharging
      PACE_GND_CTRL = 1;
      ATR_PACE_CTRL = 0;
      ATR_GND_CTRL = 0;
      VENT_PACE_CTRL = 0;
      VENT_GND_CTRL = 1;
      Z_ATR_CTRL = 0;
      Z_VENT_CTRL = 0;
      LED_ON = 0;
    state Pacing
      entry:
      %Pace Ventricle
      PACE_CHARGE_CTRL = 0;
      PACE_GND_CTRL = 1;
      ATR_PACE_CTRL = 0;
      ATR_GND_CTRL = 0;
      VENT_PACE_CTRL = 1;
      VENT_GND_CTRL = 0;
      Z_ATR_CTRL = 0;
      Z_VENT_CTRL = 0;
      LED_ON = 1;
    (default) -> VOOR.Chargin_Discharging
    VOOR.Chargin_Discharging -> VOOR.Pacing : [after(double(60000/DynamicLRL)-VPW,msec)]
    VOOR.Pacing -> VOOR.Chargin_Discharging : [after(VPW,msec)]
  InitialState -> VOO [order 2] : [Mode==2]
  InitialState -> AOO [order 1] : [Mode==1]
  InitialState -> AAI [order 3] : [Mode==3]
  InitialState -> VVI [order 4] : [Mode==4]
  InitialState -> DDDR [order 9] : [Mode==9]
  (default) -> InitialState
  InitialState -> AOOR [order 5] : [Mode==5]
  InitialState -> VOOR [order 6] : [Mode==6]
  InitialState -> AAIR [order 7] : [Mode==7]
  InitialState -> VVIR [order 8] : [Mode==8]
  data: Mode input; LRL input; VPW input; ATR_CMP_DETECT input; APW input; VENT_CMP_DETECT input; ARP input; VAmp input; AAmp input; VRP input; ATR_PACE_CTRL output; PACE_CHARGE_CTRL output; PACING_REF_PWM output; VENT_PACE_CTRL output; ATR_GND_CTRL output; PACE_GND_CTRL output; VENT_GND_CTRL output; Z_ATR_CTRL output; Z_VENT_CTRL output; LED_ON output; FRONTEND_CTRL output; HysteresisTime input; ATR_CMP_REF_PWM output; VENT_CMP_REF_PWM output; DynamicLRL input; AVD input

== matlab function simulink_group17f/Subsystem/MATLAB Function ==
  data: atrial_in input; tx output; vent_in input
function tx = build_egram_packet(atrial_in, vent_in)
%#codegen
% atrial_in : double (raw analog sample from A0)
% vent_in   : double (raw analog sample from A1)
% tx        : uint8(2x1)

    % --- Convert analog values to uint8 ---
    % You can scale these if needed. For now:
    atr_u8  = uint8( max(0, min(255, round(atrial_in))) );
    vent_u8 = uint8( max(0, min(255, round(vent_in))) );

    % --- Build 2-byte packet ---
    tx = uint8([atr_u8; vent_u8]);

end
